simulink model "et_robocon_dev_guy_out"  (R2013b)
settings: Solver=FixedStepDiscrete  SolverMode=SingleTasking  StartTime=0.0  StopTime=inf  FixedStep=balancer_ts  RelTol=1e-3
undefined symbols (not defined in the file): a_d, a_r, balancerStates_Bus0, Batt, battery_gain, battery_offset, cmd_max, current_mode_status, current_task_operation_status, DiscIntNeverNeededParam, exec_period, Init_Bus0, k_f, k_i, k_phidot, k_thetadot, lightCalib, R, STATE, TRACK_MODE_LIST, ts2, W
libraries: legonxtlib x26, simulink x11, simulink_extras x4, see_saw x1
(part 3 of 3)

== stateflow chart et_robocon_dev_guy_out/Main Controller/normal_operation_modes.line_tracking_mode ==
  state line_tracking_mode
    entry:
    desired_tail = single(2.0); %radian
    entry, during:
    PWM.tail = tail_controller(sensors.theta_T,desired_tail);
    exit:
    PWM.tail = single(0);
    state Waiting
      entry: debugFlag = uint16(400);
    state Track
      entry:
      debugFlag = uint16(401);
      bias = single(0);
      FlagSteering = single(0);
      gyroTrick = single(0);
      desired_tail = single(0); %radian
      bias_WhiteSide = lightCalib.flashingWhite + 0.3*(lightCalib.flashingBlack - lightCalib.flashingWhite);
      bias_BlackSide = lightCalib.flashingBlack - 0.45*(lightCalib.flashingBlack - lightCalib.flashingWhite);
      state preProcess [parallel]
        during:
        on every(3, tick):
        [normalizedLight, filteredLight] = processLight(sensors.light, bias,lightCalib);
        [AngleCount,EncoderReset,Angle, Distance] = analyzeEncoders(rawSensors);
        settings: executionOrder=1
      state manageRacePhases [parallel]
        settings: executionOrder=2
        state Slope
          entry:
          Speak;
          PID = single([10 0 30 0 90]');
          bias = single(0);
          FlagSteering = single(0);
          state RocketStart
            state Gyro [parallel]
              settings: executionOrder=1
              state trick
                entry: gyroTrick = single(20);
              state Normal
                entry: gyroTrick = single(0);
              (default) -> trick
              trick -> Normal : after(3*20*0.004,sec)
            state Speed [parallel]
              settings: executionOrder=2
              state slowdown
                entry: fwd = single(130)
                during:
                %fwd = fwd + single(0.005/3);
                fwd = fwd + single(1/2);
              state constantSpeed2
              (default) -> line_tracking_mode.Track.manageRacePhases.Slope.RocketStart.Speed.slowdown
              line_tracking_mode.Track.manageRacePhases.Slope.RocketStart.Speed.slowdown -> line_tracking_mode.Track.manageRacePhases.Slope.RocketStart.Speed.constantSpeed2 : [fwd >= 140]
          state BeforeRamp
            entry:
            Speak;
            bias = bias_WhiteSide;
            state slowdown1
              during:
              fwd = fwd - single(1/3)
            state constantSpeed3
            (default) -> line_tracking_mode.Track.manageRacePhases.Slope.BeforeRamp.slowdown1
            line_tracking_mode.Track.manageRacePhases.Slope.BeforeRamp.slowdown1 -> constantSpeed3 : [fwd <= 120]
          state GoDown
            entry:Speak;
            bias = bias_BlackSide;
            state speedup
              during:
              %fwd = fwd + single(1/3);
              fwd = fwd + single(1/4)
            state constantSpeed1
            (default) -> speedup
            speedup -> line_tracking_mode.Track.manageRacePhases.Slope.GoDown.constantSpeed1 : [fwd >= 130]
          state Curve
            entry:Speak;
            %PID = single([20 0 25 0 100]');
            PID = single([14 0 30 0 90]');
            bias = bias_WhiteSide;
            state slowdown
              during:
              fwd = fwd - single(1/3)
            state constantSpeed2
            (default) -> line_tracking_mode.Track.manageRacePhases.Slope.Curve.slowdown
            line_tracking_mode.Track.manageRacePhases.Slope.Curve.slowdown -> line_tracking_mode.Track.manageRacePhases.Slope.Curve.constantSpeed2 : [fwd <= 140]
          (default) -> RocketStart
          RocketStart -> BeforeRamp : [single(EncoderReset*(2*pi*4.1)/360) >= single(120)]
          BeforeRamp -> GoDown : [single(EncoderReset*(2*pi*4.1)/360) >= single(200)]
          GoDown -> Curve : [single(EncoderReset*(2*pi*4.1)/360) >= single(330)]
        state FakeRace
          entry:
          Speak;
          PID = single([14 0 20 0 70]');
          bias = single(0);
          FlagSteering = single(0);
          fwd = single(120);
        state Stop1
          entry:
          Speak;
          state slowdown
            during:
            fwd = fwd - single(4/3);
          state coast
            entry:
            PID = single([1 0 0 0 0]');
            bias = single(0);
            FlagSteering = single(1);
          state Done
            entry:
            turnLightOn;
            debugFlag = uint16(402);
            PWM.left = single(0); PWM.right = single(0);
            current_mode_status = OperationModeStatusEnum.SUCCESSFULLY_COMPLETED;
          (default) -> line_tracking_mode.Track.manageRacePhases.Stop1.slowdown
          line_tracking_mode.Track.manageRacePhases.Stop1.slowdown -> line_tracking_mode.Track.manageRacePhases.Stop1.coast : [fwd <= single(0)]
          line_tracking_mode.Track.manageRacePhases.Stop1.coast -> line_tracking_mode.Track.manageRacePhases.Stop1.Done : after(1,sec)
        state StraightSouth
          entry:
          Speak;
          PID = single([10 0 30 0 90]');
          bias = bias_BlackSide;
          FlagSteering = single(0);
          fwd = single(140);
        state Corner4
          entry:
          Speak;
          %PID = single([23 0 30 0 95]');
          % PID = single([20 0 25 0 100]');
          FlagSteering = single(0);
          state slowdown
            during:
            fwd = fwd - single(1/30);
          state constantSpeed1
            entry:
            Speak;
            during:
            PID = single([20 0 30 0 100]');
            bias = bias_WhiteSide;
          (default) -> line_tracking_mode.Track.manageRacePhases.Corner4.slowdown
          line_tracking_mode.Track.manageRacePhases.Corner4.slowdown -> line_tracking_mode.Track.manageRacePhases.Corner4.constantSpeed1 : [fwd <= 130]
        state StraightNorth
          entry:
          Speak;
          PID = single([10 0 30 0 90]');
          bias = bias_BlackSide;
          FlagSteering = single(0);
          state accelerate1
            during:
            fwd = fwd + single(1/2);
          state coast1
          (default) -> line_tracking_mode.Track.manageRacePhases.StraightNorth.accelerate1
          line_tracking_mode.Track.manageRacePhases.StraightNorth.accelerate1 -> line_tracking_mode.Track.manageRacePhases.StraightNorth.coast1 : [fwd >= 140]
        state Corner5
          entry:
          Speak;
          FlagSteering = single(0);
          state slowdown
            during:
            fwd = fwd - single(1/2);
          state constantSpeed1
            entry: PID = single([20 0 30 0 95]');
            bias = bias_BlackSide;
          (default) -> line_tracking_mode.Track.manageRacePhases.Corner5.slowdown
          line_tracking_mode.Track.manageRacePhases.Corner5.slowdown -> line_tracking_mode.Track.manageRacePhases.Corner5.constantSpeed1 : [fwd <= single(100)]
        state StraightSouthAgain
          entry:
          Speak;
          PID = single([10 0 30 0 90]');
          bias = bias_BlackSide;
          FlagSteering = single(0);
          state accelerate1
            during:
            fwd = fwd + single(1/3);
          state coast1
          (default) -> line_tracking_mode.Track.manageRacePhases.StraightSouthAgain.accelerate1
          line_tracking_mode.Track.manageRacePhases.StraightSouthAgain.accelerate1 -> line_tracking_mode.Track.manageRacePhases.StraightSouthAgain.coast1 : [fwd >= 140]
        state Corner8
          entry:
          Speak;
          PID = single([14 0 30 0 90]');
          bias = bias_WhiteSide;
          FlagSteering = single(0);
          state slowdown
            during:
            fwd = fwd - single(1/2)
          state constantSpeed1
          (default) -> line_tracking_mode.Track.manageRacePhases.Corner8.slowdown
          line_tracking_mode.Track.manageRacePhases.Corner8.slowdown -> line_tracking_mode.Track.manageRacePhases.Corner8.constantSpeed1 : [fwd <= 135]
        state StraightEast
          entry:
          Speak;
          PID = single([10 0 30 0 90]');
          bias = bias_BlackSide;
          FlagSteering = single(0);
          state accelerate1
            during:
            fwd = fwd + single(1/3);
          state coast1
          (default) -> line_tracking_mode.Track.manageRacePhases.StraightEast.accelerate1
          line_tracking_mode.Track.manageRacePhases.StraightEast.accelerate1 -> line_tracking_mode.Track.manageRacePhases.StraightEast.coast1 : [fwd >= 140]
        state Corner9
          entry:
          Speak;
          PID = single([15 0 30 0 95]');
          bias = bias_WhiteSide;
          FlagSteering = single(0);
          state slowdown
            during:
            fwd = fwd - single(1/2);
          state constantSpeed1
          (default) -> line_tracking_mode.Track.manageRacePhases.Corner9.slowdown
          line_tracking_mode.Track.manageRacePhases.Corner9.slowdown -> line_tracking_mode.Track.manageRacePhases.Corner9.constantSpeed1 : [fwd <= 100]
        state Corner10
          entry:
          Speak;
          PID = single([15 0 30 0 95]');
          bias = bias_BlackSide;
          FlagSteering = single(0);
          state slowdown1
            during:
            fwd = fwd + single(1/2)
          state constantSpeed2
          (default) -> line_tracking_mode.Track.manageRacePhases.Corner10.slowdown1
          line_tracking_mode.Track.manageRacePhases.Corner10.slowdown1 -> line_tracking_mode.Track.manageRacePhases.Corner10.constantSpeed2 : [fwd >= 130]
        state Stop
          entry:
          Speak;
          PID = single([23 0 30 0 95]');
          bias = bias_BlackSide;
          FlagSteering = single(0);
          state slowdown
            during:
            fwd = fwd - single(4/3);
          state coast
            entry:
            PID = single([1 0 0 0 0]');
            bias = single(0);
            FlagSteering = single(1);
          state Done
            entry:
            turnLightOn;
            debugFlag = uint16(402);
            PWM.left = single(0); PWM.right = single(0);
            current_mode_status = OperationModeStatusEnum.SUCCESSFULLY_COMPLETED;
          (default) -> line_tracking_mode.Track.manageRacePhases.Stop.slowdown
          line_tracking_mode.Track.manageRacePhases.Stop.slowdown -> line_tracking_mode.Track.manageRacePhases.Stop.coast : [fwd <= single(0)]
          line_tracking_mode.Track.manageRacePhases.Stop.coast -> line_tracking_mode.Track.manageRacePhases.Stop.Done : after(1,sec)
        (default) -> Slope
        FakeRace -> Stop1 : [Distance >= 3*360]
        Slope -> StraightSouth : [Distance >= single(6700)]
        StraightSouth -> Corner4 : [Distance >= single(8300)]
        Corner4 -> StraightNorth : [Distance >= single(11300)]
        StraightNorth -> Corner5 : [Distance >= single(13100)]
        Corner5 -> StraightSouthAgain : [Distance >= single(14900)]
        StraightSouthAgain -> Corner8 : [Distance >= 17200]
        Corner8 -> StraightEast : [Distance >= single(18300)]
        StraightEast -> Corner9 : [Distance >= single(19500)]
        Corner9 -> Corner10 : [Distance >= single(21900)]
        Corner10 -> Stop : [Distance >= single(25000)]
      state ApplyControl [parallel]
        during:
        on every(3, tick):  lineTrackCmd = lineTracker(normalizedLight,FlagSteering,PID,fwd)
        during:
        [PWM.left PWM.right] = balanceControl(rawSensors,lineTrackCmd,gyroTrick);
        settings: executionOrder=3
      state [normalizedLight,filteredLight] = processLight(rawLight,bias,lightcalib) [function]
      state [AngleCount,EncoderReset,Angle,Distance] = analyzeEncoders(rawSensors) [function]
      state cmd = lineTracker(lightSignal,flagSteering,PID,fwd) [function]
    state Done
      entry:
      turnLightOn;
      debugFlag = uint16(402);
      PWM.left = single(0); PWM.right = single(0);
      current_mode_status = OperationModeStatusEnum.SUCCESSFULLY_COMPLETED;
    state [leftPWM,rightPWM] = balanceControl(rawSensors,lineTrackCmd,gyroTrick) [function]
    state cmd = tail_controller(current,desired) [function]
    state turnLightOn [function]
    state Speak [function]
    (default) -> Waiting
    Waiting -> Track : [hasChangedFrom(touch,single(0)) || sensors.BT_status_in ==single(1)]
  data: rawLight function_input single size=1; bias function_input single size=1; normalizedLight function_output single size=1; filteredLight function_output single size=1; lightcalib function_input Bus: Light_Bus size=1; rawSensors function_input Bus: Sensors_Bus size=1; AngleCount function_output uint8 size=1; EncoderReset function_output single size=1; Angle function_output single size=1; Distance function_output single size=1; lightSignal function_input single size=1; flagSteering function_input single size=1; PID function_input single size=5; fwd function_input single size=1; cmd function_output; leftPWM function_output single size=1; rawSensors function_input Bus: Sensors_Bus size=1; rightPWM function_output; lineTrackCmd function_input single size=2; gyroTrick function_input single size=1; current function_input single size=1; desired function_input single size=1; cmd function_output single size=1; sensors input Bus: Sensors_Bus size=1; lightCalib data_store_memory size=1; touch input single size=1; PWM output Bus: PWM_bus size=1; debugFlag output uint16 size=1; current_mode_status data_store_memory; desired_tail local single size=1; rawSensors input Bus: Sensors_Bus size=1; lineTrackCmd local single size=2; PID local single size=5; normalizedLight local single size=1; AngleCount local uint8 size=1; EncoderReset local single size=1; Angle local single size=1; bias local single size=1; fwd local single size=1; FlagSteering local single size=1; filteredLight local single; Distance local single size=1; gyroTrick local; bias_WhiteSide local; bias_BlackSide local

== stateflow chart et_robocon_dev_guy_out/State Estimation/StateEstimation/Reset Subsystem ==
  state CheckForReset
    bind: doProcess;
    entry: doProcess;
    during: doProcess;
  (default) -> CheckForReset
  CheckForReset -> CheckForReset : [init_flag == 1]
  data: init_flag input
  events: doProcess output FUNCTION_CALL_EVENT

== stateflow chart et_robocon_dev_guy_out/Main Controller/normal_operation_modes.light_calibration_up_flashing ==
  state LightSensorCalibFlashing
    during:
    on every(3, tick): filteredLight = processLight(sensors.light);
    state WaitForBlack
      entry: debugFlag = uint16(310);
    state StoreBlack
      entry: lightCalib.flashingBlack = filteredLight;
      debugFlag = uint16(311);
      Speak;
    state WaitForWhite
      entry: debugFlag = uint16(312);
      Speak;
    state StoreWhite
      entry: lightCalib.flashingWhite = filteredLight;
      debugFlag = uint16(313);
      Speak;
      exit:
      turnLightOn;
      Speak;
    state CalibComplete
      entry:
      debugFlag = uint16(318);
      current_task_operation_status = OperationModeStatusEnum.SUCCESSFULLY_COMPLETED;
    state cmd = tail_controller(current,desired) [function]
    state Speak [function]
    state turnLightOn [function]
    state filteredLight  = processLight(rawLight) [function]
    (default) -> WaitForBlack
    WaitForBlack -> StoreBlack : [hasChangedFrom(touch,single(0))]
    StoreBlack -> WaitForWhite : after(1,sec)
    WaitForWhite -> StoreWhite : [hasChangedFrom(touch,single(0))]
    StoreWhite -> CalibComplete : after(1,sec)
  data: current function_input single size=1; desired function_input single size=1; cmd function_output single size=1; rawLight function_input single size=1; filteredLight function_output single size=1; sensors input Bus: Sensors_Bus size=1; lightCalib data_store_memory; current_task_operation_status data_store_memory; debugFlag output uint16; touch input single size=1; filteredLight local

== stateflow chart et_robocon_dev_guy_out/Main Controller ==
  state restore
  state emergency_stop
    entry:
    debugFlag = uint16(9999);
  state normal_operation_modes
    state gyro_calibration_mode
    state light_calibration_up_flashing
    state light_calibration_up
    state line_tracking_mode
    state see_saw_atomic
    state WeShouldNotBeHere
    (default) -> (junction 12) : {
        | current_mode_status = OperationModeStatusEnum.IN_PROGRESS;
        | }
    (junction 12) -> gyro_calibration_mode [order 1] : [  current_mode == OperationModeEnum.GYRO_CALIBRATION ]
    (junction 12) -> (junction 13) [order 2]
    (junction 13) -> light_calibration_up_flashing [order 1] : [ current_mode == OperationModeEnum.LIGHT_CALIBRATION_UP_FLASHING ]
    (junction 13) -> (junction 144) [order 2]
    (junction 144) -> light_calibration_up [order 1] : [ current_mode == OperationModeEnum.LIGHT_CALIBRATION_UP ]
    (junction 144) -> (junction 14) [order 2]
    (junction 14) -> line_tracking_mode [order 1] : [ current_mode == OperationModeEnum.LINE_TRACKING ]
    (junction 14) -> (junction 15) [order 2]
    (junction 15) -> see_saw_atomic [order 1] : [ current_mode == OperationModeEnum.SEE_SAW ]
    (junction 15) -> (junction 17) [order 2]
    (junction 17) -> ? [order 1] : [  current_mode == OperationModeEnum.LIMBO ]
    (junction 17) -> (junction 19) [order 1]
    (junction 19) -> ? [order 1] : [ current_mode == OperationModeEnum.LIGHT_CALIBRATION_LIMBO ]
    (junction 19) -> (junction 140) [order 1]
    (junction 140) -> ? [order 1] : [ current_mode == OperationModeEnum.SEE_SAW_PRINCESS ]
    (junction 140) -> (junction 154) [order 1]
    (junction 154) -> ? [order 1] : [ current_mode == OperationModeEnum.YOSHI ]
    (junction 154) -> (junction 99) [order 1]
    (junction 99) -> WeShouldNotBeHere
  (default) -> (junction 38) : {initFlags = Init_Bus0;BT_status_out = single(0)}
  (junction 37) -> (junction 38)
  (junction 43) -> (junction 37)
  (junction 38) -> (junction 39) : { current_mode_index = uint8( 0 ); }
  (junction 40) -> (junction 39)
  restore -> (junction 40) : [ false == touch ]
  (junction 39) -> (junction 41) : {
      | current_mode_status = OperationModeStatusEnum.NOT_STARTED;
      | }
  normal_operation_modes -> (junction 40) [order 2] : [ current_mode_status == OperationModeStatusEnum.SUCCESSFULLY_COMPLETED ]
  (junction 42) -> (junction 41)
  (junction 41) -> (junction 44) : { current_mode_index = current_mode_index + uint8( 1 ); }
  (junction 47) -> (junction 42)
  emergency_stop -> restore : [ true == touch ]
  (junction 44) -> (junction 43) [order 1] : [ numel( TRACK_MODE_LIST ) < current_mode_index ]
      | % If the "current_mode_index" has exceeded the number
      | % of elements in the list, it should "wrap" back to the start.
  (junction 44) -> (junction 45) [order 2]
  (junction 45) -> (junction 46) : {
      | current_mode = TRACK_MODE_LIST( current_mode_index );
      | }
  (junction 46) -> (junction 47) [order 1] : [  current_mode == OperationModeEnum.SKIP ]
  (junction 46) -> normal_operation_modes [order 2]
  normal_operation_modes -> emergency_stop [order 1] : [ true == fall_detection_input ]
      | {current_mode_status = OperationModeStatusEnum.ABORTED;}
  data: rawSensors input Bus: Sensors_Bus size=1; PWM output Bus: PWM_bus size=1; TRACK_MODE_LIST parameter Enum: OperationModeEnum; current_mode_index local uint8; current_mode data_store_memory; states input Bus: States_Bus size=1; fall_detection_input input boolean size=1; current_mode_status data_store_memory; sensors input Bus: Sensors_Bus size=1; lightCalib data_store_memory; debugFlag output uint16 size=1; BT_status_out output single size=1; touch input single size=1; initFlags output Bus: Init_Bus size=1; Init_Bus0 parameter Bus: Init_Bus size=1; balancerStates_Bus0 parameter Bus: Balancer_States_Bus size=1

== stateflow chart et_robocon_dev_guy_out/Main Controller/normal_operation_modes.light_calibration_up ==
  state wait
    entry:debugFlag = uint16(200);
  state MoveUp
    entry:debugFlag = uint16(201);
    PWM.tail = single(-50);
    Speak();
  state Reset
    entry:debugFlag = uint16(202);
    PWM.tail = single(0);
    initFlags.tail = single(1);
    exit:
    initFlags.tail = single(0);
    desired_tail = single(0);
    Speak;
  state Speak [function]
  state light_sensor_calibration_up
    %during, exit: PWM.tail = tail_controller(sensors.theta_T,single(1.6))
    state WaitForBlack
      entry: debugFlag = uint16(310);
    state StoreBlack
      entry: lightCalib.black = sensors.light;
      debugFlag = uint16(311);
      Speak;
    state WaitForWhite
      entry: debugFlag = uint16(312);
      Speak;
    state StoreWhite
      entry: lightCalib.white = sensors.light;
      debugFlag = uint16(313);
      Speak;
    state CalibComplete
      entry:
      Speak;
      debugFlag = uint16(318);
      current_task_operation_status = OperationModeStatusEnum.SUCCESSFULLY_COMPLETED;
    state cmd = tail_controller(current,desired) [function]
    (default) -> WaitForBlack
    WaitForBlack -> StoreBlack : [hasChangedFrom(touch,single(0))]
    StoreBlack -> WaitForWhite : after(1,sec)
    WaitForWhite -> StoreWhite : [hasChangedFrom(touch,single(0))]
    StoreWhite -> CalibComplete : after(1,sec)
  (default) -> wait
  wait -> MoveUp : [hasChangedFrom(touch,single(0))]
  MoveUp -> Reset : after(2,sec)
  Reset -> light_sensor_calibration_up : after(1,sec)
  data: current function_input single size=1; desired function_input single size=1; cmd function_output single size=1; sensors input Bus: Sensors_Bus size=1; lightCalib data_store_memory; current_task_operation_status data_store_memory; debugFlag output uint16; touch input single size=1; PWM output Bus: PWM_bus size=1; initFlags output Bus: Init_Bus size=1; desired_tail local

== stateflow chart et_robocon_dev_guy_out/Main Controller/normal_operation_modes.gyro_calibration_mode ==
  state gyro_calibration_mode
    state GyroCalibration
      entry:
      desired_tail = single(1.6);
      during, exit:
      PWM.tail = tail_controller(sensors.theta_T,desired_tail);
      state MoveTailDown
        entry:
        debugFlag = uint16(204);
        during:
        desired_tail = desired_tail + single(0.008);
      state StartCalibration
        entry:
        debugFlag = uint16(205);
        initFlags.gyroInit = single(1);
        initFlags.gyroReset = single(1);
        initFlags.theta = single(1);
      state Wait
        entry: Speak;
      state MakeNoise
        during: Speak;
      state StartCalibration1
        entry:
        debugFlag = uint16(208);
        initFlags.gyroInit = single(0);
        initFlags.gyroReset = single(0);
        initFlags.theta = single(0);
      state CalibComplete
        entry:
        debugFlag = uint16(209);
        current_task_operation_status = OperationModeStatusEnum.SUCCESSFULLY_COMPLETED;
      state cmd = tail_controller(current,desired) [function]
      state Speak [function]
      (default) -> StartCalibration
      MoveTailDown -> StartCalibration : [desired_tail >= single(1.6) ]
      StartCalibration -> Wait : [hasChangedFrom(touch,single(0))]
      Wait -> MakeNoise : after(5,sec)
      MakeNoise -> StartCalibration1 : after(0.5,sec)
      StartCalibration1 -> CalibComplete
    (default) -> GyroCalibration
  data: current function_input single size=1; desired function_input single size=1; cmd function_output single size=1; debugFlag output uint16 size=1; current_task_operation_status data_store_memory; sensors input Bus: Sensors_Bus size=1; touch input single size=1; initFlags output Bus: Init_Bus size=1; PWM output Bus: PWM_bus size=1; desired_tail local
